simulink model "InvPendOnCart"  (R2016b)
settings: Solver=ode45  StartTime=0.0  StopTime=1000  RelTol=1e-3  EnableMultiTasking=on
undefined symbols (not defined in the file or in its folder): controller, drawPendulum, P
libraries: simulink x2
settings Model: Creator=beard  LastModifiedBy=fourier
settings DataIOCC: LimitDataPoints=on  SaveFormat=Array  SignalLoggingSaveFormat=ModelDataLogs
settings OptimizationCC: ExpressionDepthLimit=2147483647  InitFltsAndDblsToZero=on  LifeSpan=inf
settings DebuggingCC: UnderspecifiedInitializationDetection=Classic  MergeDetectMultiDrivingBlocksExec=none  SolverPrmCheckMsg=warning  FcnCallInpInsideContextMsg=warning  StateNameClashWarn=warning  SFUnexpectedBacktrackingDiag=warning  SFNoUnconditionalDefaultTransitionDiag=warning  SFExecutionAtInitializationDiag=none
settings HardwareCC: ProdBitPerPointer=32  ProdBitPerSizeT=32  ProdBitPerPtrDiffT=32  ProdLargestAtomicFloat=None  ProdIntDivRoundTo=Undefined  ProdEndianess=Unspecified  ProdWordSize=32  ProdHWDeviceType=32-bit Generic
settings ModelReferenceCC: PropagateSignalLabelsOutOfModel=off
settings GRTTargetCC: TargetLangStandard=C89/C90 (ANSI)  GeneratePreprocessorConditionals=Disable all  CombineOutputUpdateFcns=off  GRTInterface=on
settings ConfigComp: CovMetricSettings=dw  CovHtmlReporting=on  CovSaveCumulativeToWorkspaceVar=on  CovSaveSingleToWorkspaceVar=on  CovExternalEMLEnable=off

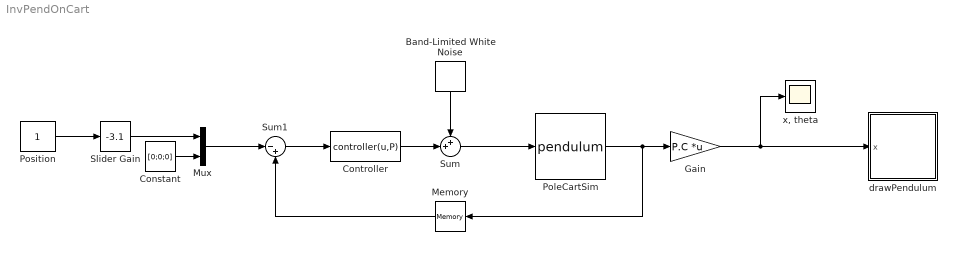
== system InvPendOnCart ==
  Band-Limited White Noise : simulink/Sources/Band-Limited White Noise  Cov=[0.1]*1  Ts=0.1  seed=[23341]
  Constant : Constant  Value=[0;0;0]
  Controller : MATLABFcn  MATLABFcn=controller(u,P)  OutputDimensions=1
  Gain : Gain  Gain=P.C  Multiplication=Matrix(K*u)
  Memory : Memory  X0=P.x0
  Mux : Mux  Inputs=2
  PoleCartSim : S-Function  FunctionName=pendulum  Parameters=P  SFunctionDeploymentMode=off  EnableBusSupport=off
      mask Display: image(imread('PendModel.jpg'))
  Position : Constant
  Slider Gain : simulink/Math Operations/Slider Gain  low=-5  gain=-3.1  high=5
  Sum : Sum  Inputs=++|
  Sum1 : Sum  Inputs=|-+
  drawPendulum : Subsystem
      mask init:
      | % drawing parameters
      | L = 2;
      | gap = 0.01;
      | width = 1.50;
      | height = 0.75;
      mask Display: image(imread('InvertedPendulum.jpg'))
  "x, theta" : Scope
  wires:
  Gain/1 -> "x, theta"/1, drawPendulum/1(x)
  Controller/1 -> Sum/2
  Band-Limited White Noise/1 -> Sum/1
  Sum/1 -> PoleCartSim/1
  PoleCartSim/1 -> Memory/1, Gain/1
  Mux/1 -> Sum1/1
  Memory/1 -> Sum1/2
  Sum1/1 -> Controller/1
  Position/1 -> Slider Gain/1
  Slider Gain/1 -> Mux/1
  Constant/1 -> Mux/2

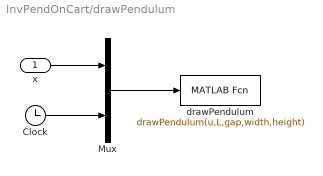
== system InvPendOnCart/drawPendulum ==
  x : Inport
  Clock : Clock
  Mux : Mux  Inputs=2
  drawPendulum : MATLABFcn  MATLABFcn=drawPendulum(u,L,gap,width,height)  OutputDimensions=0  SampleTime=0.1
  wires:
  Mux/1 -> drawPendulum/1
  x/1 -> Mux/1
  Clock/1 -> Mux/2
